simulink library "adaptlib"  (Simulink 2.20)
libraries: adaptlib x9

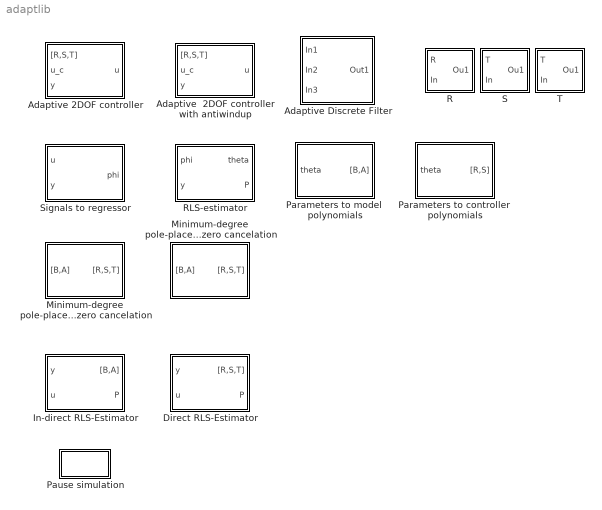
== system adaptlib ==
  Adaptive 2DOF controller : Subsystem  mask{n_r=, x_0_r=, h=}
      mask prompts: n_r "n (degree of R, S and T)"; x_0_r "Initial state (size 3n+1)"; h "Sampling period"
      mask help:
      | A two-degree-of-freedom linear controller
      |
      |   R(q)u(k) = T(q)u_c(k) - S(q)y(k)
  Adaptive  2DOF controller with antiwindup : Subsystem  mask{n_r=, ulim=, A_o=, h=}
      mask prompts: n_r "n_r (degree of R, S and T)"; ulim "Maximum control signal"; A_o "A_o (Anti windup polynomial)"; h "Sampling period"
      mask help:
      | A two-degree-of-freedom linear controller with control signal saturation and anti windup.
      |
      |   A_o(q)v(k)=T(q)u_c(k)-S(q)y(k)-(A_o(q)-R(q))u(t)
      |   u(k)=f(v(k))
  Adaptive Discrete Filter : Subsystem  mask{n_N=, n_D=, h=}
      mask prompts: n_N "n_N (degree numerator)"; n_D "n_D (degree denominator)"
      mask Display: disp(' Num(z) \n \n Den(z) \n \n u')
  Direct RLS-Estimator : Subsystem  Priority=1  mask{n_r=, theta_0=, P_0=, lambda=, A_m=, A_o=, d0=, h=}
      mask prompts: n_r "n_r (degree of R, S and T)"; theta_0 "Initial estimate"; P_0 "Initial covariance matrix"; h "Sampling period"
  In-direct RLS-Estimator : Subsystem  Priority=1  mask{m=, n=, theta_0=, P_0=, lambda=, h=}
      mask prompts: m "m (b_1 ... b_m)"; n "n (a_1 ... a_n)"; theta_0 "Initial estimate (b_1 ... b_m a_1 ... a_n]"; P_0 "Initial covariance matrix"; h "Sampling period"
  Minimum-degree pole-placement design  with zero cancelation : Subsystem  mask{n_a=, n_b=, n_r=, B_m=, A_m=, A_o=, A_r=, A_s=, h=}
      mask prompts: n_a "deg A"; n_b "deg B"; n_r "deg R"; A_r "Factor in R"; A_s "Factor in S"; h "Sampling period"
      mask help: Minimum-degree pole-placement design without zero cancellation
  Minimum-degree pole-placement design  without zero cancelation : Subsystem  mask{n_a=, n_b=, n_r=, A_o=, A_m=, A_r=, A_s=, h=}
      mask prompts: n_a "deg A"; n_b "deg B"; n_r "deg R"; A_r "Factor in R"; A_s "Factor in S"; h "Sampling period"
      mask help: Minimum-degree pole-placement design without zero cancellation
  Parameters to controller  polynomials : Subsystem  mask{n_r=}
      mask prompts: n_r "n_r (degree of R, S )"
  Parameters to model  polynomials : Subsystem  mask{m=, n=}
      mask prompts: m "m (b_1 ... b_m)"; n "n (a_1 ... a_n)"
  Pause simulation : Subsystem  mask{par=}
      mask prompts: par "Pausing time vector"
      mask help: Pauses the simulation at the times in the pausing time vector
      mask Display: disp('PAUSE')
  R : Subsystem  mask{n_D=, h=}
      mask prompts: n_D "n (degree R)"; h "Sampling period"
      mask Display:
      | plot([0.3 0.7],[0.5 0.5])
      | text(0.1,0.77,'R')
      | text(0.53,0.65,'1')
      | text(0.41,0.28,'R(z)')
  RLS-estimator : Subsystem  mask{n=, theta_0=, P_0=, lambda=, h=}
      mask prompts: n "n (number of parameters)"; theta_0 "Initial estimate"; P_0 "Initial covariance matrix"; h "Sampling period"
      mask help:
      | A discrete-time recursive least-squares estimator for a model on the form
      |
      |   y = phi'*theta
  S : Subsystem  mask{n_N=, h=}
      mask prompts: n_N "n (degree S)"; h "Sampling period"
      mask Display:
      | plot([0.3 0.7],[0.5 0.5])
      | text(0.1,0.77,'S')
      | text(0.41,0.65,'S(z)')
      | text(0.53,0.28,'1')
  Signals to regressor : Subsystem  mask{m=, n=, h=}
      mask prompts: m "m (u(t-1) ... u(t-m))"; n "n (-y(t-1) ... -y(t-n))"; h "Sampling period"
      mask help:
      | Merging of y and u to a regression vector as:
      |
      |   phi(t-1) = [u(t-1) ... u(t-m) -y(t-1) ... -y(t-n)]'
  T : Subsystem  mask{n_N=, h=}
      mask prompts: n_N "n (degree T)"; h "Sampling period"
      mask Display:
      | plot([0.3 0.7],[0.5 0.5])
      | text(0.1,0.77,'T')
      | text(0.41,0.65,'T(z)')
      | text(0.53,0.28,'1')

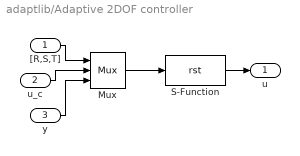
== system adaptlib/Adaptive 2DOF controller ==
  "[R,S,T]" : Inport  Port=1  PortWidth=-1  SampleTime=-1
  u_c : Inport  Port=2  PortWidth=-1  SampleTime=-1
  y : Inport  Port=3  PortWidth=-1  SampleTime=-1
  Mux : Mux  Inputs=3
  S-Function : S-Function  FunctionName=rst  Parameters=n_r,x_0_r,h  PortCounts=[]  SFunctionModules=''
  u : Outport  Port=1  InitialOutput=0
  wires:
  S-Function/1 -> u/1
  "[R,S,T]"/1 -> Mux/1
  y/1 -> Mux/3
  u_c/1 -> Mux/2
  Mux/1 -> S-Function/1

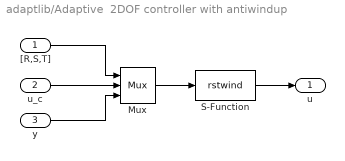
== system adaptlib/Adaptive  2DOF controller with antiwindup ==
  "[R,S,T]" : Inport  Port=1  PortWidth=-1  SampleTime=-1
  u_c : Inport  Port=2  PortWidth=-1  SampleTime=-1
  y : Inport  Port=3  PortWidth=-1  SampleTime=-1
  Mux : Mux  Inputs=3
  S-Function : S-Function  FunctionName=rstwind  Parameters=n_r,h,A_o,ulim  PortCounts=[]  SFunctionModules=''
  u : Outport  Port=1  InitialOutput=0
  wires:
  u_c/1 -> Mux/2
  S-Function/1 -> u/1
  Mux/1 -> S-Function/1
  y/1 -> Mux/3
  "[R,S,T]"/1 -> Mux/1

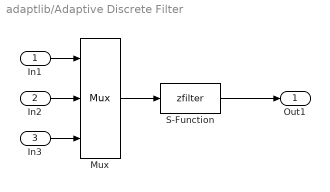
== system adaptlib/Adaptive Discrete Filter ==
  In1 : Inport  Port=1  PortWidth=-1  SampleTime=-1
  In2 : Inport  Port=2  PortWidth=-1  SampleTime=-1
  In3 : Inport  Port=3  PortWidth=-1  SampleTime=-1
  Mux : Mux  Inputs=[n_N+1 1 1]
  S-Function : S-Function  FunctionName=zfilter  Parameters=n_D,n_N,h  PortCounts=[]  SFunctionModules=''
  Out1 : Outport  Port=1
  wires:
  In1/1 -> Mux/1
  In2/1 -> Mux/2
  In3/1 -> Mux/3
  Mux/1 -> S-Function/1
  S-Function/1 -> Out1/1

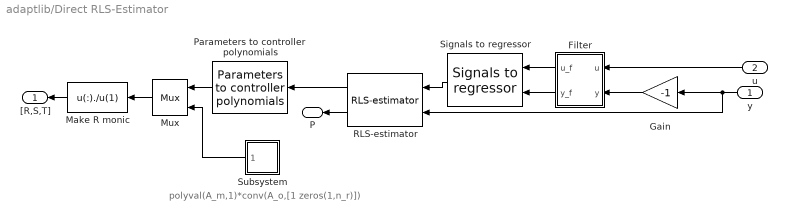
== system adaptlib/Direct RLS-Estimator ==
  note: polyval(A_m,1)*conv(A_o,[1 zeros(1,n_r)])
  y : Inport  Orientation=left  Port=1  PortWidth=-1  SampleTime=-1
  u : Inport  Orientation=left  Port=2  PortWidth=-1  SampleTime=-1
  Filter : Subsystem  Orientation=left  mask{A_m=A_m, A_o=A_o, d0=d0, h=h}
  Gain : Gain  Orientation=left  Gain=-1
  Make R monic : MATLABFcn  Orientation=left  MATLABFcn=u(:)./u(1)  OutputWidth=3*(n_r+1)
  Mux : Mux  Orientation=left  Inputs=2
  Parameters to controller  polynomials : adaptlib/Parameters to controller  polynomials  Orientation=left  n_r=n_r
  RLS-estimator : adaptlib/RLS-estimator  Orientation=left  n=2*(n_r+1)  theta_0=theta_0  P_0=P_0  lambda=lambda  h=h
  Signals to regressor : adaptlib/Signals to regressor  Orientation=left  m=n_r+1  n=n_r+1  h=h
  Subsystem : Subsystem  Orientation=left
      mask Display: disp('T')
  "[R,S,T]" : Outport  Orientation=left  Port=1  InitialOutput=0
  P : Outport  Orientation=left  Port=2  InitialOutput=0
  wires:
  Subsystem/1(Out1) -> Mux/2
  Parameters to controller  polynomials/1 -> Mux/1
  RLS-estimator/1 -> Parameters to controller  polynomials/1
  RLS-estimator/2 -> P/1
  Signals to regressor/1 -> RLS-estimator/1
  Filter/2(y_f) -> Signals to regressor/2
  Filter/1(u_f) -> Signals to regressor/1
  y/1 -> RLS-estimator/2, Gain/1
  u/1 -> Filter/1(u)
  Gain/1 -> Filter/2(y)
  Mux/1 -> Make R monic/1
  Make R monic/1 -> "[R,S,T]"/1

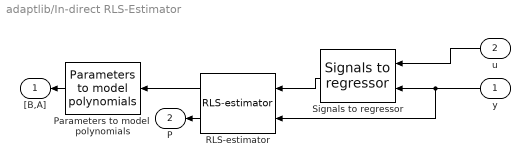
== system adaptlib/In-direct RLS-Estimator ==
  y : Inport  Orientation=left  Port=1  PortWidth=-1  SampleTime=-1
  u : Inport  Orientation=left  Port=2  PortWidth=-1  SampleTime=-1
  Parameters to model  polynomials : adaptlib/Parameters to model  polynomials  Orientation=left  m=m  n=n
  RLS-estimator : adaptlib/RLS-estimator  Orientation=left  n=m+n  theta_0=theta_0  P_0=P_0  lambda=lambda  h=h
  Signals to regressor : adaptlib/Signals to regressor  Orientation=left  m=m  n=n  h=h
  "[B,A]" : Outport  Orientation=left  Port=1  InitialOutput=0
  P : Outport  Orientation=left  Port=2  InitialOutput=0
  wires:
  Parameters to model  polynomials/1 -> "[B,A]"/1
  RLS-estimator/1 -> Parameters to model  polynomials/1
  RLS-estimator/2 -> P/1
  y/1 -> Signals to regressor/2, RLS-estimator/2
  Signals to regressor/1 -> RLS-estimator/1
  u/1 -> Signals to regressor/1

== system adaptlib/Minimum-degree pole-placement design  with zero cancelation ==
  "[B,A]" : Inport  Port=1  PortWidth=-1  SampleTime=-1
  S-Function : S-Function  FunctionName=zdesign  Parameters=n_a,n_b,n_r,B_m,A_m,A_o,A_r,A_s,h  PortCounts=[]  SFunctionModules=''
  "[R,S,T]" : Outport  Port=1
  wires:
  S-Function/1 -> "[R,S,T]"/1
  "[B,A]"/1 -> S-Function/1

== system adaptlib/Minimum-degree pole-placement design  without zero cancelation ==
  "[B,A]" : Inport  Port=1  PortWidth=-1  SampleTime=-1
  S-Function : S-Function  FunctionName=nzdesign  Parameters=n_a,n_b,n_r,A_m,A_o,A_r,A_s,h  PortCounts=[]  SFunctionModules=''
  "[R,S,T]" : Outport  Port=1
  wires:
  "[B,A]"/1 -> S-Function/1
  S-Function/1 -> "[R,S,T]"/1

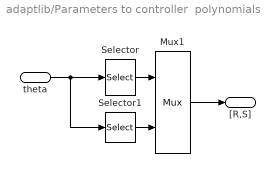
== system adaptlib/Parameters to controller  polynomials ==
  theta : Inport  Port=1  PortWidth=-1  SampleTime=-1
  Mux1 : Mux  Inputs=2
  Selector : Selector  Elements=[1 : n_r+1]  InputPortWidth=2*(n_r+1)
  Selector1 : Selector  Elements="[n_r+2 :  2*(n_r+1)]"  InputPortWidth=2*(n_r+1)
  "[R,S]" : Outport  Port=1  InitialOutput=0
  wires:
  theta/1 -> Selector1/1, Selector/1
  Selector/1 -> Mux1/1
  Mux1/1 -> "[R,S]"/1
  Selector1/1 -> Mux1/2

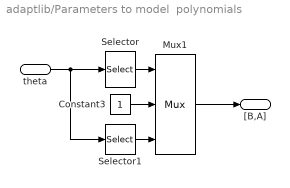
== system adaptlib/Parameters to model  polynomials ==
  theta : Inport  Port=1  PortWidth=-1  SampleTime=-1
  Constant3 : Constant  Value=1
  Mux1 : Mux  Inputs=3
  Selector : Selector  Elements=[1 : m]  InputPortWidth=m+n
  Selector1 : Selector  Elements="[m+1 :  m+n]"  InputPortWidth=m+n
  "[B,A]" : Outport  Port=1  InitialOutput=0
  wires:
  Constant3/1 -> Mux1/2
  Mux1/1 -> "[B,A]"/1
  Selector/1 -> Mux1/1
  Selector1/1 -> Mux1/3
  theta/1 -> Selector/1, Selector1/1

== system adaptlib/Pause simulation ==
  Pause simulation : S-Function  FunctionName=pausesim  Parameters=par  PortCounts=[]  SFunctionModules=''

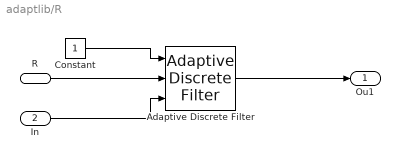
== system adaptlib/R ==
  R : Inport  Port=1  PortWidth=-1  SampleTime=-1
  In : Inport  Port=2  PortWidth=-1  SampleTime=-1
  Adaptive Discrete Filter : adaptlib/Adaptive Discrete Filter  n_N=0  n_D=n_D  h=h
  Constant : Constant  Value=1
  Ou1 : Outport  Port=1
  wires:
  Constant/1 -> Adaptive Discrete Filter/1
  Adaptive Discrete Filter/1 -> Ou1/1
  In/1 -> Adaptive Discrete Filter/3
  R/1 -> Adaptive Discrete Filter/2

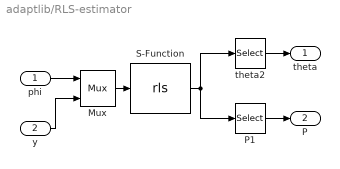
== system adaptlib/RLS-estimator ==
  phi : Inport  Port=1  PortWidth=-1  SampleTime=-1
  y : Inport  Port=2  PortWidth=-1  SampleTime=-1
  Mux : Mux  Inputs=2
  P1 : Selector  Elements=[n+1:n+n^2]  InputPortWidth=n+n^2
  S-Function : S-Function  FunctionName=rls  Parameters=n,theta_0,P_0,lambda,h  PortCounts=[]  SFunctionModules=''
  theta2 : Selector  Elements=[1:n]  InputPortWidth=n+n^2
  theta : Outport  Port=1  InitialOutput=0
  P : Outport  Port=2  InitialOutput=0
  wires:
  phi/1 -> Mux/1
  y/1 -> Mux/2
  S-Function/1 -> theta2/1, P1/1
  theta2/1 -> theta/1
  P1/1 -> P/1
  Mux/1 -> S-Function/1

== system adaptlib/S ==
  T : Inport  Port=1  PortWidth=-1  SampleTime=-1
  In : Inport  Port=2  PortWidth=-1  SampleTime=-1
  Adaptive Discrete Filter : adaptlib/Adaptive Discrete Filter  n_N=n_N  n_D=0  h=h
  Constant : Constant  Value=1
  Ou1 : Outport  Port=1
  wires:
  In/1 -> Adaptive Discrete Filter/3
  Adaptive Discrete Filter/1 -> Ou1/1
  Constant/1 -> Adaptive Discrete Filter/2
  T/1 -> Adaptive Discrete Filter/1

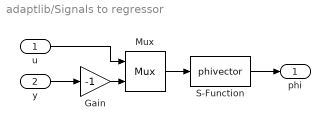
== system adaptlib/Signals to regressor ==
  u : Inport  Port=1  PortWidth=-1  SampleTime=-1
  y : Inport  Port=2  PortWidth=-1  SampleTime=-1
  Gain : Gain  Gain=-1
  Mux : Mux  Inputs=2
  S-Function : S-Function  FunctionName=phivector  Parameters=m,n,h  PortCounts=[]  SFunctionModules=''
  phi : Outport  Port=1
  wires:
  y/1 -> Gain/1
  Gain/1 -> Mux/2
  u/1 -> Mux/1
  S-Function/1 -> phi/1
  Mux/1 -> S-Function/1

== system adaptlib/T ==
  T : Inport  Port=1  PortWidth=-1  SampleTime=-1
  In : Inport  Port=2  PortWidth=-1  SampleTime=-1
  Adaptive Discrete Filter : adaptlib/Adaptive Discrete Filter  n_N=n_N  n_D=0  h=h
  Constant : Constant  Value=1
  Ou1 : Outport  Port=1
  wires:
  T/1 -> Adaptive Discrete Filter/1
  Constant/1 -> Adaptive Discrete Filter/2
  Adaptive Discrete Filter/1 -> Ou1/1
  In/1 -> Adaptive Discrete Filter/3

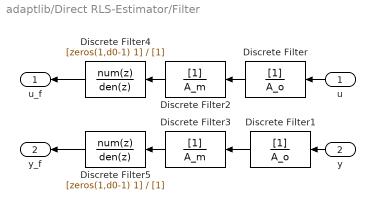
== system adaptlib/Direct RLS-Estimator/Filter ==
  u : Inport  Orientation=left  Port=1  PortWidth=-1  SampleTime=-1
  y : Inport  Orientation=left  Port=2  PortWidth=-1  SampleTime=-1
  Discrete Filter : DiscreteFilter  Orientation=left  Numerator=[1]  Denominator=A_o  SampleTime=h
  Discrete Filter1 : DiscreteFilter  Orientation=left  Numerator=[1]  Denominator=A_o  SampleTime=h
  Discrete Filter2 : DiscreteFilter  Orientation=left  Numerator=[1]  Denominator=A_m  SampleTime=h
  Discrete Filter3 : DiscreteFilter  Orientation=left  Numerator=[1]  Denominator=A_m  SampleTime=h
  Discrete Filter4 : DiscreteFilter  Orientation=left  Numerator=[zeros(1,d0-1) 1]  Denominator=[1]  SampleTime=h
  Discrete Filter5 : DiscreteFilter  Orientation=left  Numerator=[zeros(1,d0-1) 1]  Denominator=[1]  SampleTime=h
  u_f : Outport  Orientation=left  Port=1  InitialOutput=0
  y_f : Outport  Orientation=left  Port=2  InitialOutput=0
  wires:
  Discrete Filter1/1 -> Discrete Filter3/1
  Discrete Filter/1 -> Discrete Filter2/1
  y/1 -> Discrete Filter1/1
  u/1 -> Discrete Filter/1
  Discrete Filter3/1 -> Discrete Filter5/1
  Discrete Filter5/1 -> y_f/1
  Discrete Filter2/1 -> Discrete Filter4/1
  Discrete Filter4/1 -> u_f/1

== system adaptlib/Direct RLS-Estimator/Subsystem ==
  Constant : Constant  Orientation=left  Value=polyval(A_m,1)*conv(A_o,[1 zeros(1,n_r)])
  Out1 : Outport  Orientation=left  Port=1
  wires:
  Constant/1 -> Out1/1
